simulink library "quant_xcorr_lib"  (Simulink 7.1)
libraries: xbsIndex_r4 x48, quant_xcorr_lib x36
settings Model: Creator=Administrator  LastModifiedBy=Jonathan Weintroub

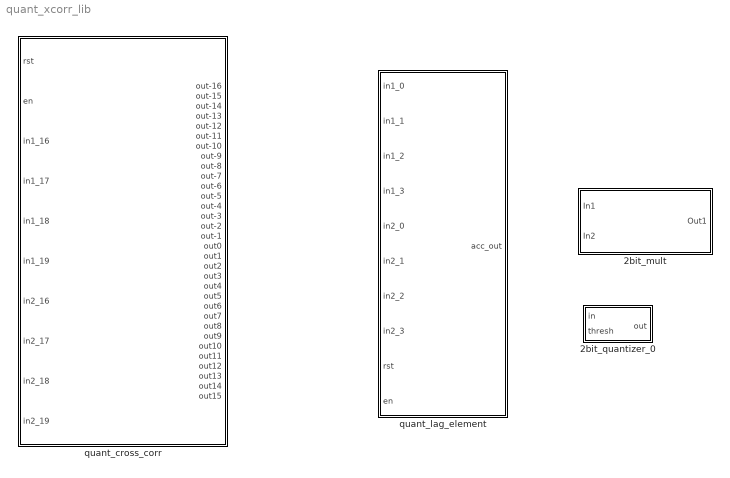
== system quant_xcorr_lib ==
  2bit_mult : Subsystem
  2bit_quantizer_0 : Subsystem
  quant_cross_corr : Subsystem  mask(quant_cross_corr){ants=2, demuxr2=2, bits=2, lags=8, range=positive and negative lags}
      mask prompts: ants "Antennas:"; demuxr2 "Demux (2^?):"; bits "Bitwidth:"; lags "Lags (in multiples of demux):"
      mask init:
      | quant_cross_corr_init(gcb,...
      |     'ants', ants,...
      |     'demuxr2', demuxr2,...
      |     'bits', bits,...
      |     'lags', lags,...
      |     'range', range);
      settings: AttributesFormatString=antennas=2, demux=4, lags=32
      mask StyleString: edit,edit,edit,edit,popup(positive and negative lags|positive lags only)
  quant_lag_element : Subsystem  mask(quant_lag_element){demux=2, lag=6}
      mask prompts: demux "Demux (2^?):"; lag "Lag Number:"
      mask init:
      | quant_lag_element_init(gcb,...
      |     'demux', demux, 'lag', lag);
      settings: AttributesFormatString=demux=4, lag=1

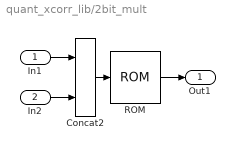
== system quant_xcorr_lib/2bit_mult ==
  In1 : Inport  OutDataType=sfix(16)  OutScaling=2^0
  In2 : Inport  Port=2  OutDataType=sfix(16)  OutScaling=2^0
  Concat2 : xbsIndex_r4/Concat  num_inputs=2  dbl_ovrd=off  block_type=concat
      settings: block_version=10.1.3
  ROM : xbsIndex_r4/ROM  depth=16  initVector=[1; 3; -1; -3; 3; 9; -3; -9; -1; -3; 1; 3; -3; -9; 3; 9]  distributed_mem=Distributed memory  rst=off  init_reg=0  en=off  latency=1  arith_type="Signed  (2's comp)"  n_bits=5  bin_pt=0  dbl_ovrd=off  optimize=Area  use_rpm=off  block_type=sprom
      settings: xl_area=[0, 0, 0, 0, 0, 0, 0]  block_version=10.1.3
  Out1 : Outport  OutDataType=sfix(16)  OutScaling=2^0
  wires:
  In2/1 -> Concat2/2
  ROM/1 -> Out1/1
  In1/1 -> Concat2/1
  Concat2/1 -> ROM/1

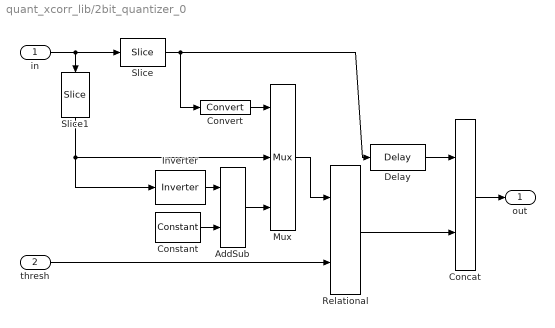
== system quant_xcorr_lib/2bit_quantizer_0 ==
  in : Inport  OutDataType=sfix(16)  OutScaling=2^0
  thresh : Inport  Port=2  OutDataType=sfix(16)  OutScaling=2^0
  AddSub : xbsIndex_r4/AddSub  mode=Addition  use_carryin=off  use_carryout=off  en=off  latency=0  precision=Full  arith_type=Unsigned  n_bits=8  bin_pt=2  quantization=Truncate  overflow=Wrap  dbl_ovrd=off  use_behavioral_HDL=on  pipelined=off  use_rpm=on  hw_selection=Fabric  block_type=addsub
      settings: xl_area=[0, 0, 0, 0, 0, 0, 0]  block_version=10.1.3
  Concat : xbsIndex_r4/Concat  num_inputs=2  dbl_ovrd=off  block_type=concat
      settings: block_version=10.1.3
  Constant : xbsIndex_r4/Constant  arith_type=Unsigned  const=1  n_bits=7  bin_pt=0  explicit_period=on  period=1  equ=P=C  opselect=C  inp2=PCIN>>17  opr=+  inp1=P  carry=CIN  dbl_ovrd=off  block_type=constant
  Convert : xbsIndex_r4/Convert  arith_type=Boolean  n_bits=8  bin_pt=6  quantization=Truncate  overflow=Wrap  latency=0  dbl_ovrd=off  pipeline=off  block_type=convert
      settings: xl_area=[0, 0, 0, 0, 0, 0, 0]  block_version=10.1.3
  Delay : xbsIndex_r4/Delay  en=off  latency=1  dbl_ovrd=off  reg_retiming=off  block_type=delay
      settings: xl_area=[0, 0, 0, 0, 0, 0, 0]
  Inverter : xbsIndex_r4/Inverter  en=off  latency=0  dbl_ovrd=off  block_type=inv
      settings: xl_area=[0, 0, 0, 0, 0, 0, 0]
  Mux : xbsIndex_r4/Mux  inputs=2  en=off  latency=0  precision=Full  arith_type="Signed  (2's comp)"  n_bits=8  bin_pt=2  quantization=Truncate  overflow=Wrap  dbl_ovrd=off  block_type=mux
      settings: xl_area=[0, 0, 0, 0, 0, 0, 0]
  Relational : xbsIndex_r4/Relational  mode=a>=b  en=off  latency=1  dbl_ovrd=off  block_type=relational
      settings: xl_area=[0, 0, 0, 0, 0, 0, 0]  block_version=10.1.3
  Slice : xbsIndex_r4/Slice  nbits=1  boolean_output=off  mode=Upper Bit Location + Width  bit1=0  base1=MSB of Input  bit0=0  base0=LSB of Input  dbl_ovrd=off  block_type=slice
      settings: infoedit="Extracts a given range of bits from each input sample and presents it at the output.  The output type is ordinarily unsigned with binary point at zero, but can be Boolean when the slice is one bit wide.<P><P>Hardware notes: In hardware this block costs nothing."  block_version=10.1.3
  Slice1 : xbsIndex_r4/Slice  Orientation=down  nbits=7  boolean_output=off  mode=Upper Bit Location + Width  bit1=-1  base1=MSB of Input  bit0=0  base0=LSB of Input  dbl_ovrd=off  block_type=slice
      settings: infoedit="Extracts a given range of bits from each input sample and presents it at the output.  The output type is ordinarily unsigned with binary point at zero, but can be Boolean when the slice is one bit wide.<P><P>Hardware notes: In hardware this block costs nothing."  block_version=10.1.3
  out : Outport  OutDataType=sfix(16)  OutScaling=2^0
  wires:
  in/1 -> Slice/1, Slice1/1
  Concat/1 -> out/1
  Slice/1 -> Delay/1, Convert/1
  Relational/1 -> Concat/2
  thresh/1 -> Relational/2
  Delay/1 -> Concat/1
  Inverter/1 -> AddSub/1
  Constant/1 -> AddSub/2
  Convert/1 -> Mux/1
  Mux/1 -> Relational/1
  Slice1/1 -> Mux/2, Inverter/1
  AddSub/1 -> Mux/3

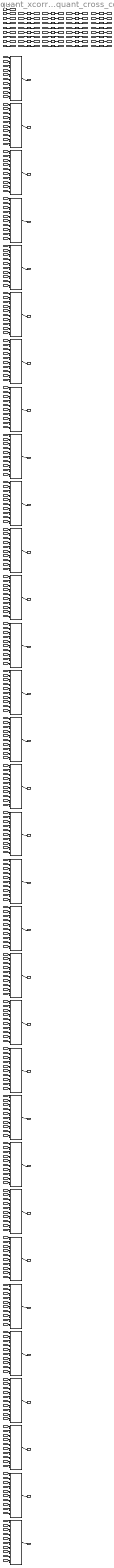
== system quant_xcorr_lib/quant_cross_corr ==
  rst : Inport  OutDataType=sfix(16)  OutScaling=2^0
  en : Inport  Port=2  OutDataType=sfix(16)  OutScaling=2^0
  in1_16 : Inport  Port=3  OutDataType=sfix(16)  OutScaling=2^0
  in1_17 : Inport  Port=4  OutDataType=sfix(16)  OutScaling=2^0
  in1_18 : Inport  Port=5  OutDataType=sfix(16)  OutScaling=2^0
  in1_19 : Inport  Port=6  OutDataType=sfix(16)  OutScaling=2^0
  in2_16 : Inport  Port=7  OutDataType=sfix(16)  OutScaling=2^0
  in2_17 : Inport  Port=8  OutDataType=sfix(16)  OutScaling=2^0
  in2_18 : Inport  Port=9  OutDataType=sfix(16)  OutScaling=2^0
  in2_19 : Inport  Port=10  OutDataType=sfix(16)  OutScaling=2^0
  in1_16_del{1..4} (4 alike) : xbsIndex_r4/Delay  en=off  latency=1  dbl_ovrd=off  reg_retiming=off  block_type=delay
      settings: xl_area=[0, 0, 0, 0, 0, 0, 0]
  in1_17_del{1..4} (4 alike) : xbsIndex_r4/Delay  en=off  latency=1  dbl_ovrd=off  reg_retiming=off  block_type=delay
      settings: xl_area=[0, 0, 0, 0, 0, 0, 0]
  in1_18_del{1..4} (4 alike) : xbsIndex_r4/Delay  en=off  latency=1  dbl_ovrd=off  reg_retiming=off  block_type=delay
      settings: xl_area=[0, 0, 0, 0, 0, 0, 0]
  in1_19_del{1..4} (4 alike) : xbsIndex_r4/Delay  en=off  latency=1  dbl_ovrd=off  reg_retiming=off  block_type=delay
      settings: xl_area=[0, 0, 0, 0, 0, 0, 0]
  in2_16_del{1..4} (4 alike) : xbsIndex_r4/Delay  en=off  latency=1  dbl_ovrd=off  reg_retiming=off  block_type=delay
      settings: xl_area=[0, 0, 0, 0, 0, 0, 0]
  in2_17_del{1..4} (4 alike) : xbsIndex_r4/Delay  en=off  latency=1  dbl_ovrd=off  reg_retiming=off  block_type=delay
      settings: xl_area=[0, 0, 0, 0, 0, 0, 0]
  in2_18_del{1..4} (4 alike) : xbsIndex_r4/Delay  en=off  latency=1  dbl_ovrd=off  reg_retiming=off  block_type=delay
      settings: xl_area=[0, 0, 0, 0, 0, 0, 0]
  in2_19_del{1..4} (4 alike) : xbsIndex_r4/Delay  en=off  latency=1  dbl_ovrd=off  reg_retiming=off  block_type=delay
      settings: xl_area=[0, 0, 0, 0, 0, 0, 0]
  lag-1 : quant_xcorr_lib/quant_lag_element  SystemSampleTime=-1  demux=2  lag=-1
      settings: AttributesFormatString=demux=4, lag=-1
  lag-10 : quant_xcorr_lib/quant_lag_element  SystemSampleTime=-1  demux=2  lag=-10
      settings: AttributesFormatString=demux=4, lag=-10
  lag-11 : quant_xcorr_lib/quant_lag_element  SystemSampleTime=-1  demux=2  lag=-11
      settings: AttributesFormatString=demux=4, lag=-11
  lag-12 : quant_xcorr_lib/quant_lag_element  SystemSampleTime=-1  demux=2  lag=-12
      settings: AttributesFormatString=demux=4, lag=-12
  lag-13 : quant_xcorr_lib/quant_lag_element  SystemSampleTime=-1  demux=2  lag=-13
      settings: AttributesFormatString=demux=4, lag=-13
  lag-14 : quant_xcorr_lib/quant_lag_element  SystemSampleTime=-1  demux=2  lag=-14
      settings: AttributesFormatString=demux=4, lag=-14
  lag-15 : quant_xcorr_lib/quant_lag_element  SystemSampleTime=-1  demux=2  lag=-15
      settings: AttributesFormatString=demux=4, lag=-15
  lag-16 : quant_xcorr_lib/quant_lag_element  SystemSampleTime=-1  demux=2  lag=-16
      settings: AttributesFormatString=demux=4, lag=-16
  lag-2 : quant_xcorr_lib/quant_lag_element  SystemSampleTime=-1  demux=2  lag=-2
      settings: AttributesFormatString=demux=4, lag=-2
  lag-3 : quant_xcorr_lib/quant_lag_element  SystemSampleTime=-1  demux=2  lag=-3
      settings: AttributesFormatString=demux=4, lag=-3
  lag-4 : quant_xcorr_lib/quant_lag_element  SystemSampleTime=-1  demux=2  lag=-4
      settings: AttributesFormatString=demux=4, lag=-4
  lag-5 : quant_xcorr_lib/quant_lag_element  SystemSampleTime=-1  demux=2  lag=-5
      settings: AttributesFormatString=demux=4, lag=-5
  lag-6 : quant_xcorr_lib/quant_lag_element  SystemSampleTime=-1  demux=2  lag=-6
      settings: AttributesFormatString=demux=4, lag=-6
  lag-7 : quant_xcorr_lib/quant_lag_element  SystemSampleTime=-1  demux=2  lag=-7
      settings: AttributesFormatString=demux=4, lag=-7
  lag-8 : quant_xcorr_lib/quant_lag_element  SystemSampleTime=-1  demux=2  lag=-8
      settings: AttributesFormatString=demux=4, lag=-8
  lag-9 : quant_xcorr_lib/quant_lag_element  SystemSampleTime=-1  demux=2  lag=-9
      settings: AttributesFormatString=demux=4, lag=-9
  lag0 : quant_xcorr_lib/quant_lag_element  SystemSampleTime=-1  demux=2  lag=0
      settings: AttributesFormatString=demux=4, lag=0
  lag1 : quant_xcorr_lib/quant_lag_element  SystemSampleTime=-1  demux=2  lag=1
      settings: AttributesFormatString=demux=4, lag=1
  lag10 : quant_xcorr_lib/quant_lag_element  SystemSampleTime=-1  demux=2  lag=10
      settings: AttributesFormatString=demux=4, lag=10
  lag11 : quant_xcorr_lib/quant_lag_element  SystemSampleTime=-1  demux=2  lag=11
      settings: AttributesFormatString=demux=4, lag=11
  lag12 : quant_xcorr_lib/quant_lag_element  SystemSampleTime=-1  demux=2  lag=12
      settings: AttributesFormatString=demux=4, lag=12
  lag13 : quant_xcorr_lib/quant_lag_element  SystemSampleTime=-1  demux=2  lag=13
      settings: AttributesFormatString=demux=4, lag=13
  lag14 : quant_xcorr_lib/quant_lag_element  SystemSampleTime=-1  demux=2  lag=14
      settings: AttributesFormatString=demux=4, lag=14
  lag15 : quant_xcorr_lib/quant_lag_element  SystemSampleTime=-1  demux=2  lag=15
      settings: AttributesFormatString=demux=4, lag=15
  lag2 : quant_xcorr_lib/quant_lag_element  SystemSampleTime=-1  demux=2  lag=2
      settings: AttributesFormatString=demux=4, lag=2
  lag3 : quant_xcorr_lib/quant_lag_element  SystemSampleTime=-1  demux=2  lag=3
      settings: AttributesFormatString=demux=4, lag=3
  lag4 : quant_xcorr_lib/quant_lag_element  SystemSampleTime=-1  demux=2  lag=4
      settings: AttributesFormatString=demux=4, lag=4
  lag5 : quant_xcorr_lib/quant_lag_element  SystemSampleTime=-1  demux=2  lag=5
      settings: AttributesFormatString=demux=4, lag=5
  lag6 : quant_xcorr_lib/quant_lag_element  SystemSampleTime=-1  demux=2  lag=6
      settings: AttributesFormatString=demux=4, lag=6
  lag7 : quant_xcorr_lib/quant_lag_element  SystemSampleTime=-1  demux=2  lag=7
      settings: AttributesFormatString=demux=4, lag=7
  lag8 : quant_xcorr_lib/quant_lag_element  SystemSampleTime=-1  demux=2  lag=8
      settings: AttributesFormatString=demux=4, lag=8
  lag9 : quant_xcorr_lib/quant_lag_element  SystemSampleTime=-1  demux=2  lag=9
      settings: AttributesFormatString=demux=4, lag=9
  out-16 : Outport  OutDataType=sfix(16)  OutScaling=2^0
  out-15 : Outport  Port=2  OutDataType=sfix(16)  OutScaling=2^0
  out-14 : Outport  Port=3  OutDataType=sfix(16)  OutScaling=2^0
  out-13 : Outport  Port=4  OutDataType=sfix(16)  OutScaling=2^0
  out-12 : Outport  Port=5  OutDataType=sfix(16)  OutScaling=2^0
  out-11 : Outport  Port=6  OutDataType=sfix(16)  OutScaling=2^0
  out-10 : Outport  Port=7  OutDataType=sfix(16)  OutScaling=2^0
  out-9 : Outport  Port=8  OutDataType=sfix(16)  OutScaling=2^0
  out-8 : Outport  Port=9  OutDataType=sfix(16)  OutScaling=2^0
  out-7 : Outport  Port=10  OutDataType=sfix(16)  OutScaling=2^0
  out-6 : Outport  Port=11  OutDataType=sfix(16)  OutScaling=2^0
  out-5 : Outport  Port=12  OutDataType=sfix(16)  OutScaling=2^0
  out-4 : Outport  Port=13  OutDataType=sfix(16)  OutScaling=2^0
  out-3 : Outport  Port=14  OutDataType=sfix(16)  OutScaling=2^0
  out-2 : Outport  Port=15  OutDataType=sfix(16)  OutScaling=2^0
  out-1 : Outport  Port=16  OutDataType=sfix(16)  OutScaling=2^0
  out0 : Outport  Port=17  OutDataType=sfix(16)  OutScaling=2^0
  out1 : Outport  Port=18  OutDataType=sfix(16)  OutScaling=2^0
  out2 : Outport  Port=19  OutDataType=sfix(16)  OutScaling=2^0
  out3 : Outport  Port=20  OutDataType=sfix(16)  OutScaling=2^0
  out4 : Outport  Port=21  OutDataType=sfix(16)  OutScaling=2^0
  out5 : Outport  Port=22  OutDataType=sfix(16)  OutScaling=2^0
  out6 : Outport  Port=23  OutDataType=sfix(16)  OutScaling=2^0
  out7 : Outport  Port=24  OutDataType=sfix(16)  OutScaling=2^0
  out8 : Outport  Port=25  OutDataType=sfix(16)  OutScaling=2^0
  out9 : Outport  Port=26  OutDataType=sfix(16)  OutScaling=2^0
  out10 : Outport  Port=27  OutDataType=sfix(16)  OutScaling=2^0
  out11 : Outport  Port=28  OutDataType=sfix(16)  OutScaling=2^0
  out12 : Outport  Port=29  OutDataType=sfix(16)  OutScaling=2^0
  out13 : Outport  Port=30  OutDataType=sfix(16)  OutScaling=2^0
  out14 : Outport  Port=31  OutDataType=sfix(16)  OutScaling=2^0
  out15 : Outport  Port=32  OutDataType=sfix(16)  OutScaling=2^0
  wires:
  rst/1 -> [reset]
  en/1 -> [enable]
  in1_16/1 -> [in1_16]
  [in1_16] -> in1_16_del1/1
  in1_16_del1/1 -> [in1_12]
  [in1_12] -> in1_16_del2/1
  in1_16_del2/1 -> [in1_8]
  [in1_8] -> in1_16_del3/1
  in1_16_del3/1 -> [in1_4]
  [in1_4] -> in1_16_del4/1
  in1_16_del4/1 -> [in1_0]
  in1_17/1 -> [in1_17]
  [in1_17] -> in1_17_del1/1
  in1_17_del1/1 -> [in1_13]
  [in1_13] -> in1_17_del2/1
  in1_17_del2/1 -> [in1_9]
  [in1_9] -> in1_17_del3/1
  in1_17_del3/1 -> [in1_5]
  [in1_5] -> in1_17_del4/1
  in1_17_del4/1 -> [in1_1]
  in1_18/1 -> [in1_18]
  [in1_18] -> in1_18_del1/1
  in1_18_del1/1 -> [in1_14]
  [in1_14] -> in1_18_del2/1
  in1_18_del2/1 -> [in1_10]
  [in1_10] -> in1_18_del3/1
  in1_18_del3/1 -> [in1_6]
  [in1_6] -> in1_18_del4/1
  in1_18_del4/1 -> [in1_2]
  in1_19/1 -> [in1_19]
  [in1_19] -> in1_19_del1/1
  in1_19_del1/1 -> [in1_15]
  [in1_15] -> in1_19_del2/1
  in1_19_del2/1 -> [in1_11]
  [in1_11] -> in1_19_del3/1
  in1_19_del3/1 -> [in1_7]
  [in1_7] -> in1_19_del4/1
  in1_19_del4/1 -> [in1_3]
  in2_16/1 -> [in2_16]
  [in2_16] -> in2_16_del1/1
  in2_16_del1/1 -> [in2_12]
  [in2_12] -> in2_16_del2/1
  in2_16_del2/1 -> [in2_8]
  [in2_8] -> in2_16_del3/1
  in2_16_del3/1 -> [in2_4]
  [in2_4] -> in2_16_del4/1
  in2_16_del4/1 -> [in2_0]
  in2_17/1 -> [in2_17]
  [in2_17] -> in2_17_del1/1
  in2_17_del1/1 -> [in2_13]
  [in2_13] -> in2_17_del2/1
  in2_17_del2/1 -> [in2_9]
  [in2_9] -> in2_17_del3/1
  in2_17_del3/1 -> [in2_5]
  [in2_5] -> in2_17_del4/1
  in2_17_del4/1 -> [in2_1]
  in2_18/1 -> [in2_18]
  [in2_18] -> in2_18_del1/1
  in2_18_del1/1 -> [in2_14]
  [in2_14] -> in2_18_del2/1
  in2_18_del2/1 -> [in2_10]
  [in2_10] -> in2_18_del3/1
  in2_18_del3/1 -> [in2_6]
  [in2_6] -> in2_18_del4/1
  in2_18_del4/1 -> [in2_2]
  in2_19/1 -> [in2_19]
  [in2_19] -> in2_19_del1/1
  in2_19_del1/1 -> [in2_15]
  [in2_15] -> in2_19_del2/1
  in2_19_del2/1 -> [in2_11]
  [in2_11] -> in2_19_del3/1
  in2_19_del3/1 -> [in2_7]
  [in2_7] -> in2_19_del4/1
  in2_19_del4/1 -> [in2_3]
  [in1_16] -> lag-16/1
  [in1_17] -> lag-16/2
  [in1_18] -> lag-16/3
  [in1_19] -> lag-16/4
  [in2_0] -> lag-16/5
  [in2_1] -> lag-16/6
  [in2_2] -> lag-16/7
  [in2_3] -> lag-16/8
  [reset] -> lag-16/9
  [enable] -> lag-16/10
  lag-16/1 -> out-16/1
  [in1_15] -> lag-15/1
  [in1_16] -> lag-15/2
  [in1_17] -> lag-15/3
  [in1_18] -> lag-15/4
  [in2_0] -> lag-15/5
  [in2_1] -> lag-15/6
  [in2_2] -> lag-15/7
  [in2_3] -> lag-15/8
  [reset] -> lag-15/9
  [enable] -> lag-15/10
  lag-15/1 -> out-15/1
  [in1_14] -> lag-14/1
  [in1_15] -> lag-14/2
  [in1_16] -> lag-14/3
  [in1_17] -> lag-14/4
  [in2_0] -> lag-14/5
  [in2_1] -> lag-14/6
  [in2_2] -> lag-14/7
  [in2_3] -> lag-14/8
  [reset] -> lag-14/9
  [enable] -> lag-14/10
  lag-14/1 -> out-14/1
  [in1_13] -> lag-13/1
  [in1_14] -> lag-13/2
  [in1_15] -> lag-13/3
  [in1_16] -> lag-13/4
  [in2_0] -> lag-13/5
  [in2_1] -> lag-13/6
  [in2_2] -> lag-13/7
  [in2_3] -> lag-13/8
  [reset] -> lag-13/9
  [enable] -> lag-13/10
  lag-13/1 -> out-13/1
  [in1_12] -> lag-12/1
  [in1_13] -> lag-12/2
  [in1_14] -> lag-12/3
  [in1_15] -> lag-12/4
  [in2_0] -> lag-12/5
  [in2_1] -> lag-12/6
  [in2_2] -> lag-12/7
  [in2_3] -> lag-12/8
  [reset] -> lag-12/9
  [enable] -> lag-12/10
  lag-12/1 -> out-12/1
  [in1_11] -> lag-11/1
  [in1_12] -> lag-11/2
  [in1_13] -> lag-11/3
  [in1_14] -> lag-11/4
  [in2_0] -> lag-11/5
  [in2_1] -> lag-11/6
  [in2_2] -> lag-11/7
  [in2_3] -> lag-11/8
  [reset] -> lag-11/9
  [enable] -> lag-11/10
  lag-11/1 -> out-11/1
  [in1_10] -> lag-10/1
  [in1_11] -> lag-10/2
  [in1_12] -> lag-10/3
  [in1_13] -> lag-10/4
  [in2_0] -> lag-10/5
  [in2_1] -> lag-10/6
  [in2_2] -> lag-10/7
  [in2_3] -> lag-10/8
  [reset] -> lag-10/9
  [enable] -> lag-10/10
  lag-10/1 -> out-10/1
  [in1_9] -> lag-9/1
  [in1_10] -> lag-9/2
  [in1_11] -> lag-9/3
  [in1_12] -> lag-9/4
  [in2_0] -> lag-9/5
  [in2_1] -> lag-9/6
  [in2_2] -> lag-9/7
  [in2_3] -> lag-9/8
  [reset] -> lag-9/9
  [enable] -> lag-9/10
  lag-9/1 -> out-9/1
  [in1_8] -> lag-8/1
  [in1_9] -> lag-8/2
  [in1_10] -> lag-8/3
  [in1_11] -> lag-8/4
  [in2_0] -> lag-8/5
  [in2_1] -> lag-8/6
  [in2_2] -> lag-8/7
  [in2_3] -> lag-8/8
  [reset] -> lag-8/9
  [enable] -> lag-8/10
  lag-8/1 -> out-8/1
  [in1_7] -> lag-7/1
  [in1_8] -> lag-7/2
  [in1_9] -> lag-7/3
  [in1_10] -> lag-7/4
  [in2_0] -> lag-7/5
  [in2_1] -> lag-7/6
  [in2_2] -> lag-7/7
  [in2_3] -> lag-7/8
  [reset] -> lag-7/9
  [enable] -> lag-7/10
  lag-7/1 -> out-7/1
  [in1_6] -> lag-6/1
  [in1_7] -> lag-6/2
  [in1_8] -> lag-6/3
  [in1_9] -> lag-6/4
  [in2_0] -> lag-6/5
  [in2_1] -> lag-6/6
  [in2_2] -> lag-6/7
  [in2_3] -> lag-6/8
  [reset] -> lag-6/9
  [enable] -> lag-6/10
  lag-6/1 -> out-6/1
  [in1_5] -> lag-5/1
  [in1_6] -> lag-5/2
  [in1_7] -> lag-5/3
  [in1_8] -> lag-5/4
  [in2_0] -> lag-5/5
  [in2_1] -> lag-5/6
  [in2_2] -> lag-5/7
  [in2_3] -> lag-5/8
  [reset] -> lag-5/9
  [enable] -> lag-5/10
  lag-5/1 -> out-5/1
  [in1_4] -> lag-4/1
  [in1_5] -> lag-4/2
  [in1_6] -> lag-4/3
  [in1_7] -> lag-4/4
  [in2_0] -> lag-4/5
  [in2_1] -> lag-4/6
  [in2_2] -> lag-4/7
  [in2_3] -> lag-4/8
  [reset] -> lag-4/9
  [enable] -> lag-4/10
  lag-4/1 -> out-4/1
  [in1_3] -> lag-3/1
  [in1_4] -> lag-3/2
  [in1_5] -> lag-3/3
  [in1_6] -> lag-3/4
  [in2_0] -> lag-3/5
  [in2_1] -> lag-3/6
  [in2_2] -> lag-3/7
  [in2_3] -> lag-3/8
  [reset] -> lag-3/9
  [enable] -> lag-3/10
  lag-3/1 -> out-3/1
  [in1_2] -> lag-2/1
  [in1_3] -> lag-2/2
  [in1_4] -> lag-2/3
  [in1_5] -> lag-2/4
  [in2_0] -> lag-2/5
  [in2_1] -> lag-2/6
  [in2_2] -> lag-2/7
  [in2_3] -> lag-2/8
  [reset] -> lag-2/9
  [enable] -> lag-2/10
  lag-2/1 -> out-2/1
  [in1_1] -> lag-1/1
  [in1_2] -> lag-1/2
  [in1_3] -> lag-1/3
  [in1_4] -> lag-1/4
  [in2_0] -> lag-1/5
  [in2_1] -> lag-1/6
  [in2_2] -> lag-1/7
  [in2_3] -> lag-1/8
  [reset] -> lag-1/9
  [enable] -> lag-1/10
  lag-1/1 -> out-1/1
  [in1_0] -> lag0/1
  [in1_1] -> lag0/2
  [in1_2] -> lag0/3
  [in1_3] -> lag0/4
  [in2_0] -> lag0/5
  [in2_1] -> lag0/6
  [in2_2] -> lag0/7
  [in2_3] -> lag0/8
  [reset] -> lag0/9
  [enable] -> lag0/10
  lag0/1 -> out0/1
  [in1_0] -> lag1/1
  [in1_1] -> lag1/2
  [in1_2] -> lag1/3
  [in1_3] -> lag1/4
  [in2_1] -> lag1/5
  [in2_2] -> lag1/6
  [in2_3] -> lag1/7
  [in2_4] -> lag1/8
  [reset] -> lag1/9
  [enable] -> lag1/10
  lag1/1 -> out1/1
  [in1_0] -> lag2/1
  [in1_1] -> lag2/2
  [in1_2] -> lag2/3
  [in1_3] -> lag2/4
  [in2_2] -> lag2/5
  [in2_3] -> lag2/6
  [in2_4] -> lag2/7
  [in2_5] -> lag2/8
  [reset] -> lag2/9
  [enable] -> lag2/10
  lag2/1 -> out2/1
  [in1_0] -> lag3/1
  [in1_1] -> lag3/2
  [in1_2] -> lag3/3
  [in1_3] -> lag3/4
  [in2_3] -> lag3/5
  [in2_4] -> lag3/6
  [in2_5] -> lag3/7
  [in2_6] -> lag3/8
  [reset] -> lag3/9
  [enable] -> lag3/10
  lag3/1 -> out3/1
  [in1_0] -> lag4/1
  [in1_1] -> lag4/2
  [in1_2] -> lag4/3
  [in1_3] -> lag4/4
  [in2_4] -> lag4/5
  [in2_5] -> lag4/6
  [in2_6] -> lag4/7
  [in2_7] -> lag4/8
  [reset] -> lag4/9
  [enable] -> lag4/10
  lag4/1 -> out4/1
  [in1_0] -> lag5/1
  [in1_1] -> lag5/2
  [in1_2] -> lag5/3
  [in1_3] -> lag5/4
  [in2_5] -> lag5/5
  [in2_6] -> lag5/6
  [in2_7] -> lag5/7
  [in2_8] -> lag5/8
  [reset] -> lag5/9
  [enable] -> lag5/10
  lag5/1 -> out5/1
  [in1_0] -> lag6/1
  [in1_1] -> lag6/2
  [in1_2] -> lag6/3
  [in1_3] -> lag6/4
  [in2_6] -> lag6/5
  [in2_7] -> lag6/6
  [in2_8] -> lag6/7
  [in2_9] -> lag6/8
  [reset] -> lag6/9
  [enable] -> lag6/10
  lag6/1 -> out6/1
  [in1_0] -> lag7/1
  [in1_1] -> lag7/2
  [in1_2] -> lag7/3
  [in1_3] -> lag7/4
  [in2_7] -> lag7/5
  [in2_8] -> lag7/6
  [in2_9] -> lag7/7
  [in2_10] -> lag7/8
  [reset] -> lag7/9
  [enable] -> lag7/10
  lag7/1 -> out7/1
  [in1_0] -> lag8/1
  [in1_1] -> lag8/2
  [in1_2] -> lag8/3
  [in1_3] -> lag8/4
  [in2_8] -> lag8/5
  [in2_9] -> lag8/6
  [in2_10] -> lag8/7
  [in2_11] -> lag8/8
  [reset] -> lag8/9
  [enable] -> lag8/10
  lag8/1 -> out8/1
  [in1_0] -> lag9/1
  [in1_1] -> lag9/2
  [in1_2] -> lag9/3
  [in1_3] -> lag9/4
  [in2_9] -> lag9/5
  [in2_10] -> lag9/6
  [in2_11] -> lag9/7
  [in2_12] -> lag9/8
  [reset] -> lag9/9
  [enable] -> lag9/10
  lag9/1 -> out9/1
  [in1_0] -> lag10/1
  [in1_1] -> lag10/2
  [in1_2] -> lag10/3
  [in1_3] -> lag10/4
  [in2_10] -> lag10/5
  [in2_11] -> lag10/6
  [in2_12] -> lag10/7
  [in2_13] -> lag10/8
  [reset] -> lag10/9
  [enable] -> lag10/10
  lag10/1 -> out10/1
  [in1_0] -> lag11/1
  [in1_1] -> lag11/2
  [in1_2] -> lag11/3
  [in1_3] -> lag11/4
  [in2_11] -> lag11/5
  [in2_12] -> lag11/6
  [in2_13] -> lag11/7
  [in2_14] -> lag11/8
  [reset] -> lag11/9
  [enable] -> lag11/10
  lag11/1 -> out11/1
  [in1_0] -> lag12/1
  [in1_1] -> lag12/2
  [in1_2] -> lag12/3
  [in1_3] -> lag12/4
  [in2_12] -> lag12/5
  [in2_13] -> lag12/6
  [in2_14] -> lag12/7
  [in2_15] -> lag12/8
  [reset] -> lag12/9
  [enable] -> lag12/10
  lag12/1 -> out12/1
  [in1_0] -> lag13/1
  [in1_1] -> lag13/2
  [in1_2] -> lag13/3
  [in1_3] -> lag13/4
  [in2_13] -> lag13/5
  [in2_14] -> lag13/6
  [in2_15] -> lag13/7
  [in2_16] -> lag13/8
  [reset] -> lag13/9
  [enable] -> lag13/10
  lag13/1 -> out13/1
  [in1_0] -> lag14/1
  [in1_1] -> lag14/2
  [in1_2] -> lag14/3
  [in1_3] -> lag14/4
  [in2_14] -> lag14/5
  [in2_15] -> lag14/6
  [in2_16] -> lag14/7
  [in2_17] -> lag14/8
  [reset] -> lag14/9
  [enable] -> lag14/10
  lag14/1 -> out14/1
  [in1_0] -> lag15/1
  [in1_1] -> lag15/2
  [in1_2] -> lag15/3
  [in1_3] -> lag15/4
  [in2_15] -> lag15/5
  [in2_16] -> lag15/6
  [in2_17] -> lag15/7
  [in2_18] -> lag15/8
  [reset] -> lag15/9
  [enable] -> lag15/10
  lag15/1 -> out15/1

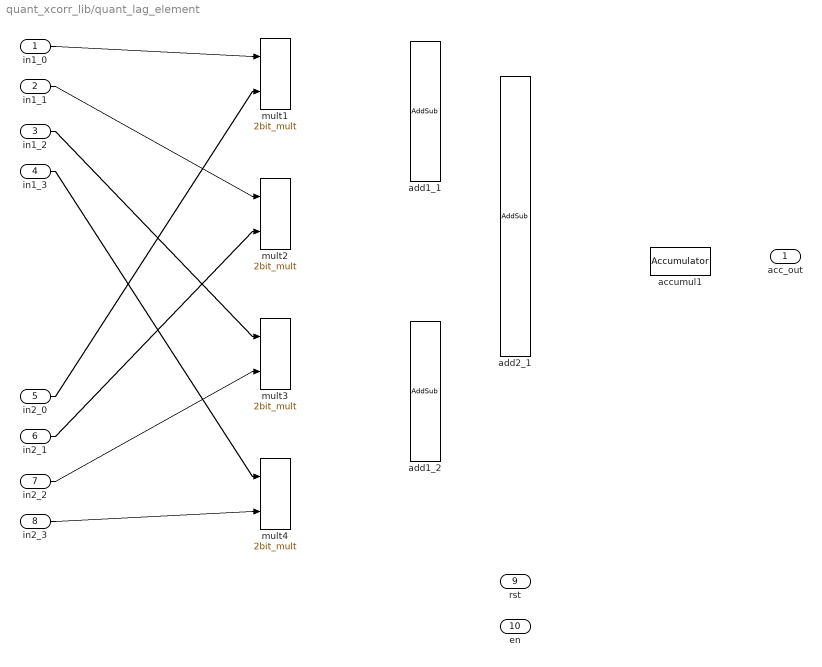
== system quant_xcorr_lib/quant_lag_element ==
  in1_0 : Inport  OutDataType=sfix(16)  OutScaling=2^0
  in1_1 : Inport  Port=2  OutDataType=sfix(16)  OutScaling=2^0
  in1_2 : Inport  Port=3  OutDataType=sfix(16)  OutScaling=2^0
  in1_3 : Inport  Port=4  OutDataType=sfix(16)  OutScaling=2^0
  in2_0 : Inport  Port=5  OutDataType=sfix(16)  OutScaling=2^0
  in2_1 : Inport  Port=6  OutDataType=sfix(16)  OutScaling=2^0
  in2_2 : Inport  Port=7  OutDataType=sfix(16)  OutScaling=2^0
  in2_3 : Inport  Port=8  OutDataType=sfix(16)  OutScaling=2^0
  rst : Inport  Port=9  OutDataType=sfix(16)  OutScaling=2^0
  en : Inport  Port=10  OutDataType=sfix(16)  OutScaling=2^0
  accumul1 : xbsIndex_r4/Accumulator  operation=Add  n_bits=32  overflow=Saturate  scale=1  rst=on  hasbypass=off  en=on  dbl_ovrd=off  use_behavioral_HDL=on  implementation=Fabric  block_type=accum
      settings: infoedit="Adder or subtractor-based accumulator.   Output type and binary point position match the input.<P><P>Hardware notes: When \"Reinitialize with input 'b' on reset\" is selected, the accumulator is forced to run at the system rate even if the input 'b' is running at a slower rate."  xl_area=[0, 0, 0, 0, 0, 0, 0]  block_version=10.1.3
  add1_1 : xbsIndex_r4/AddSub  mode=Addition  use_carryin=off  use_carryout=off  en=off  latency=1  precision=Full  arith_type=Unsigned  n_bits=8  bin_pt=2  quantization=Truncate  overflow=Wrap  dbl_ovrd=off  use_behavioral_HDL=on  pipelined=on  use_rpm=on  hw_selection=Fabric  block_type=addsub
      settings: xl_area=[0, 0, 0, 0, 0, 0, 0]  block_version=10.1.3
  add1_2 : xbsIndex_r4/AddSub  mode=Addition  use_carryin=off  use_carryout=off  en=off  latency=1  precision=Full  arith_type=Unsigned  n_bits=8  bin_pt=2  quantization=Truncate  overflow=Wrap  dbl_ovrd=off  use_behavioral_HDL=on  pipelined=on  use_rpm=on  hw_selection=Fabric  block_type=addsub
      settings: xl_area=[0, 0, 0, 0, 0, 0, 0]  block_version=10.1.3
  add2_1 : xbsIndex_r4/AddSub  mode=Addition  use_carryin=off  use_carryout=off  en=off  latency=1  precision=Full  arith_type=Unsigned  n_bits=8  bin_pt=2  quantization=Truncate  overflow=Wrap  dbl_ovrd=off  use_behavioral_HDL=on  pipelined=on  use_rpm=on  hw_selection=Fabric  block_type=addsub
      settings: xl_area=[0, 0, 0, 0, 0, 0, 0]  block_version=10.1.3
  mult{1..4} (4 alike) : quant_xcorr_lib/2bit_mult  SystemSampleTime=-1
  acc_out : Outport  OutDataType=sfix(16)  OutScaling=2^0
  wires:
  in1_0/1 -> mult1/1
  in2_0/1 -> mult1/2
  in1_1/1 -> mult2/1
  in2_1/1 -> mult2/2
  in1_2/1 -> mult3/1
  in2_2/1 -> mult3/2
  in1_3/1 -> mult4/1
  in2_3/1 -> mult4/2
